simulink model "stateflow_23a"  (R2023a)
settings: Solver=VariableStepAuto  StartTime=0.0  StopTime=10.0  RelTol=1e-3
settings Model: Creator=uditpant  LastModifiedBy=uditpant

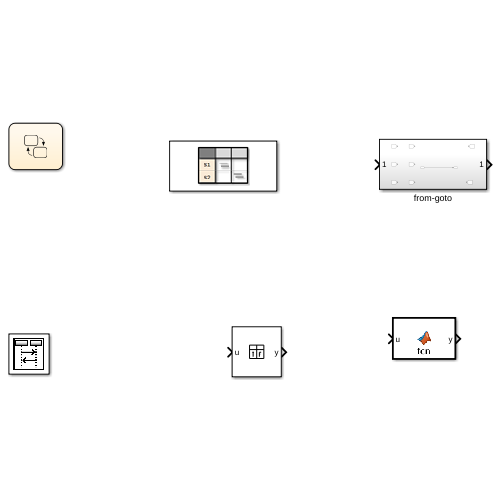
[thumbnail: Simulink's stored preview of the top-level diagram]
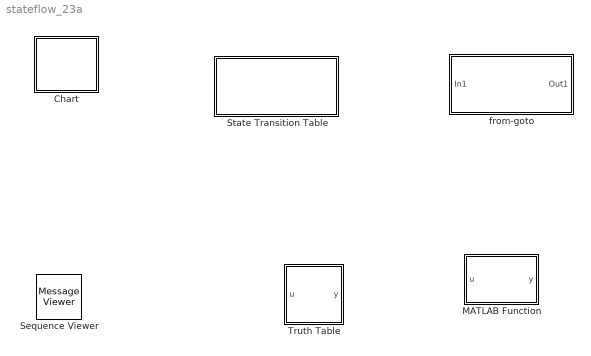
== system stateflow_23a ==
  Chart : Stateflow chart  TreatAsAtomicUnit=on
  MATLAB Function : MATLAB Function  TreatAsAtomicUnit=on
  Sequence Viewer : MessageViewer
  State Transition Table : State Transition Table  TreatAsAtomicUnit=on
  Truth Table : Truth Table  TreatAsAtomicUnit=on
  from-goto : Subsystem

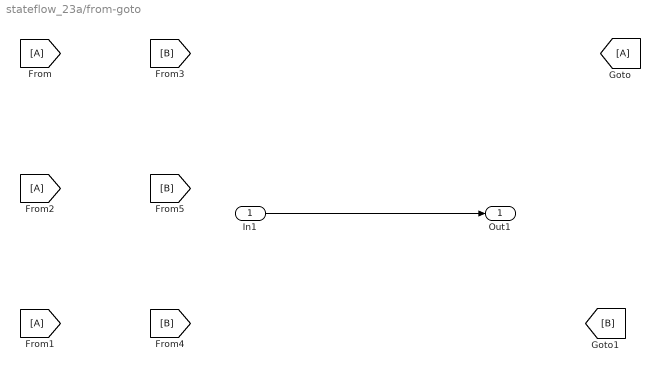
== system stateflow_23a/from-goto ==
  In1 : Inport
  From : From
  From1 : From
  From2 : From
  Goto : Goto
  Out1 : Outport
  wires:
  In1/1 -> Out1/1

== matlab function stateflow_23a/MATLAB Function ==
  data: u input; y output
function y = fcn(u)

y = u;

== matlab function stateflow_23a/Truth Table ==
  data: u input; y output
function y = fcn(u)

aVarTruthTableCondition_1 = false;
aVarTruthTableCondition_2 = false;


% Example condition 1

aVarTruthTableCondition_1 = logical(u >= 0);

% Example condition 2

aVarTruthTableCondition_2 = logical(u ^ 2 <= 1);

if (aVarTruthTableCondition_1 && aVarTruthTableCondition_2)
    aFcnTruthTableAction_1();
elseif (~aVarTruthTableCondition_1 && ~aVarTruthTableCondition_2)
    aFcnTruthTableAction_1();
else % Default
    aFcnTruthTableAction_2();
end

function aFcnTruthTableAction_1()

% Example action 1 called from D1 & D2 column in condition table

y = u;

function aFcnTruthTableAction_2()

% Example action 2 called from D3 column in condition table

y = 1 / u;

== stateflow chart stateflow_23a/Chart ==

== stateflow chart stateflow_23a/State Transition Table ==
  state state1
  state state2
  (default) -> state1
  state1 -> state2
